simulink subsystem "sub_encoder_metros_R"  (R2023b)
settings: Solver=VariableStepAuto  StartTime=0.0  StopTime=10.0  RelTol=1e-3
libraries: arduinosensorlib x2
settings Model: Creator=ricfe  LastModifiedBy=ricfe

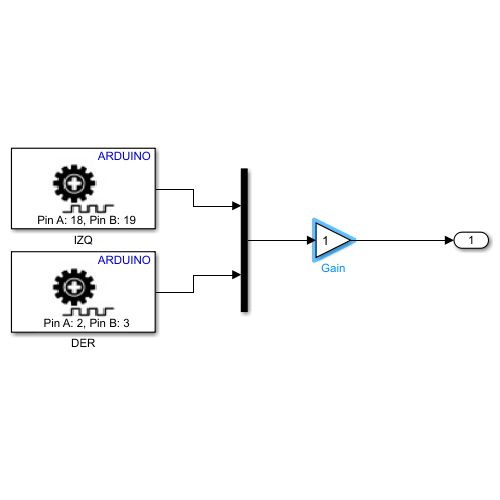
[thumbnail: Simulink's stored preview of the top-level diagram]
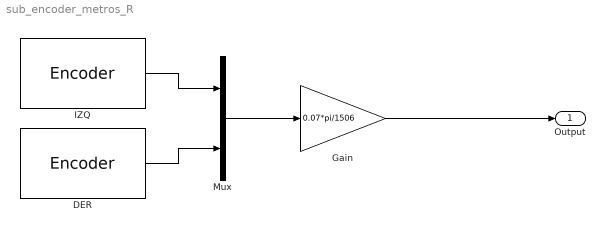
== system sub_encoder_metros_R ==
  DER : arduinosensorlib/Encoder  InputA=2  InputB=3  Mode=No reset  SampleTime=-1
  Gain : Gain  Gain=0.07*pi/1506  ParamDataTypeStr=double
  IZQ : arduinosensorlib/Encoder  InputA=18  InputB=19  Mode=No reset  SampleTime=-1
  Mux : Mux  Inputs=2
  Output : Outport
  wires:
  DER/1 -> Mux/2
  IZQ/1 -> Mux/1
  Mux/1 -> Gain/1
  Gain/1 -> Output/1
